simulink model "Multiplier"  (R2017b)
settings: Solver=ode45  StartTime=0.0  StopTime=10.0  RelTol=1e-3  EnableMultiTasking=on
libraries: hdlsllib x17
(part 1 of 3)
settings Model: Creator=you.r  LastModifiedBy=Ray
settings DataIOCC: LimitDataPoints=on  SaveFormat=Array
settings OptimizationCC: LifeSpan=inf
settings DebuggingCC: SolverPrmCheckMsg=warning  SFUnexpectedBacktrackingDiag=warning  SFNoUnconditionalDefaultTransitionDiag=warning  SFExecutionAtInitializationDiag=none
settings HardwareCC: ProdBitPerPointer=32  ProdBitPerSizeT=32  ProdBitPerPtrDiffT=32  ProdLargestAtomicFloat=None  ProdIntDivRoundTo=Undefined  ProdEndianess=Unspecified  ProdWordSize=32  ProdHWDeviceType=32-bit Generic
settings ModelReferenceCC: PropagateSignalLabelsOutOfModel=off
settings CodeAppCC: StateflowObjectComments=on
settings GRTTargetCC: TargetLangStandard=C89/C90 (ANSI)  GeneratePreprocessorConditionals=Disable all
settings ConfigComp: CovMetricSettings=dw  CovHtmlReporting=on  CovSaveCumulativeToWorkspaceVar=on  CovSaveSingleToWorkspaceVar=on  CovExternalEMLEnable=off  CovSFcnEnable=off

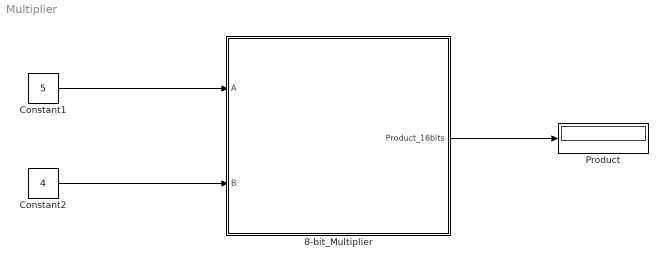
== system Multiplier ==
  8-bit_Multiplier : Subsystem
  Constant1 : Constant  Value=5  OutDataTypeStr=uint8  SampleTime=100
  Constant2 : Constant  Value=4  OutDataTypeStr=uint8  SampleTime=1
  Product : Display
  wires:
  8-bit_Multiplier/1(Product_16bits) -> Product/1
  Constant1/1 -> 8-bit_Multiplier/1(A)
  Constant2/1 -> 8-bit_Multiplier/2(B)

== system Multiplier/8-bit_Multiplier ==
  A : Inport  OutDataTypeStr=uint8
  B : Inport  Port=2  OutDataTypeStr=uint8
  Bit Concat : Subsystem
  Multiplier : Subsystem
  X Slicer : Subsystem
  X Slicer1 : Subsystem
  Product_16bits : Outport
  wires:
  B/1 -> X Slicer1/1(X)
  A/1 -> X Slicer/1(X)
  Bit Concat/1(out) -> Product_16bits/1
  Multiplier/1(P0) -> Bit Concat/16(In16)
  Multiplier/2(P1) -> Bit Concat/15(In15)
  Multiplier/3(P2) -> Bit Concat/14(In14)
  Multiplier/4(P3) -> Bit Concat/13(In13)
  Multiplier/5(P4) -> Bit Concat/12(In12)
  Multiplier/6(P5) -> Bit Concat/11(In11)
  Multiplier/7(P6) -> Bit Concat/10(In10)
  Multiplier/8(P7) -> Bit Concat/9(In9)
  Multiplier/9(P15) -> Bit Concat/1(In1)
  Multiplier/10(P14) -> Bit Concat/2(In2)
  Multiplier/11(P13) -> Bit Concat/3(In3)
  Multiplier/12(P12) -> Bit Concat/4(In4)
  Multiplier/13(P11) -> Bit Concat/5(In5)
  Multiplier/14(P10) -> Bit Concat/6(In6)
  Multiplier/15(P9) -> Bit Concat/7(In7)
  Multiplier/16(P8) -> Bit Concat/8(In8)
  X Slicer/1(Y0) -> Multiplier/8(A0)
  X Slicer/2(Y1) -> Multiplier/7(A1)
  X Slicer/3(Y2) -> Multiplier/6(A2)
  X Slicer/4(Y3) -> Multiplier/5(A3)
  X Slicer/5(Y4) -> Multiplier/4(A4)
  X Slicer/6(Y5) -> Multiplier/3(A5)
  X Slicer/7(Y6) -> Multiplier/2(A6)
  X Slicer/8(Y7) -> Multiplier/1(A7)
  X Slicer1/1(Y0) -> Multiplier/9(B0)
  X Slicer1/2(Y1) -> Multiplier/10(B1)
  X Slicer1/3(Y2) -> Multiplier/11(B2)
  X Slicer1/4(Y3) -> Multiplier/12(B3)
  X Slicer1/5(Y4) -> Multiplier/13(B4)
  X Slicer1/6(Y5) -> Multiplier/14(B5)
  X Slicer1/7(Y6) -> Multiplier/15(B6)
  X Slicer1/8(Y7) -> Multiplier/16(B7)

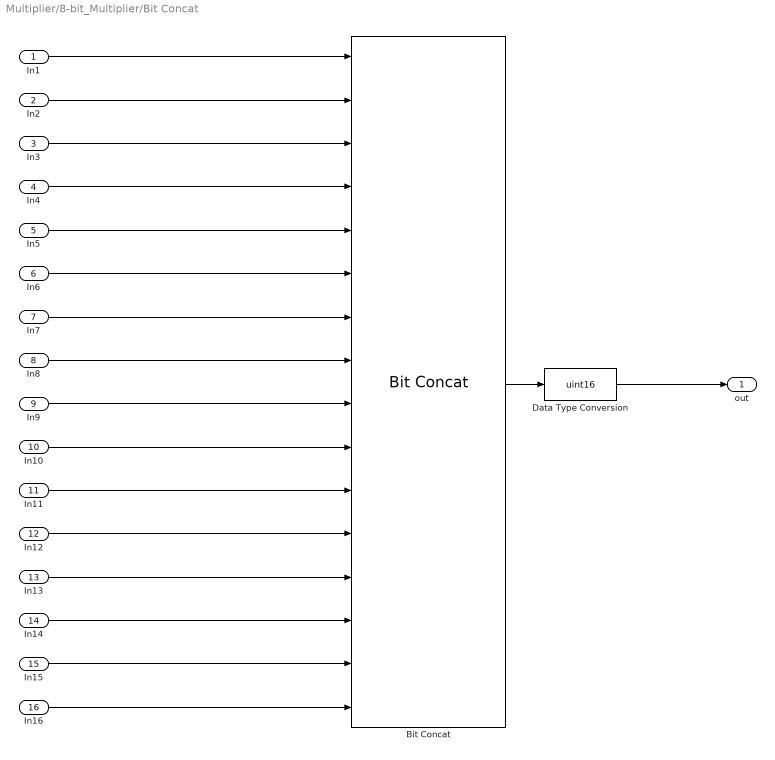
== system Multiplier/8-bit_Multiplier/Bit Concat ==
  In1 : Inport
  In2 : Inport  Port=2
  In3 : Inport  Port=3
  In4 : Inport  Port=4
  In5 : Inport  Port=5
  In6 : Inport  Port=6
  In7 : Inport  Port=7
  In8 : Inport  Port=8
  In9 : Inport  Port=9
  In10 : Inport  Port=10
  In11 : Inport  Port=11
  In12 : Inport  Port=12
  In13 : Inport  Port=13
  In14 : Inport  Port=14
  In15 : Inport  Port=15
  In16 : Inport  Port=16
  Bit Concat : hdlsllib/Logic and Bit Operations/Bit Concat  numInputs=16
      settings: SourceProductName=HDL Coder  SourceProductBaseCode=HD
  Data Type Conversion : DataTypeConversion  OutDataTypeStr=uint16
  out : Outport
  wires:
  Data Type Conversion/1 -> out/1
  Bit Concat/1 -> Data Type Conversion/1
  In13/1 -> Bit Concat/13
  In9/1 -> Bit Concat/9
  In10/1 -> Bit Concat/10
  In15/1 -> Bit Concat/15
  In1/1 -> Bit Concat/1
  In7/1 -> Bit Concat/7
  In2/1 -> Bit Concat/2
  In5/1 -> Bit Concat/5
  In11/1 -> Bit Concat/11
  In14/1 -> Bit Concat/14
  In12/1 -> Bit Concat/12
  In3/1 -> Bit Concat/3
  In4/1 -> Bit Concat/4
  In6/1 -> Bit Concat/6
  In16/1 -> Bit Concat/16
  In8/1 -> Bit Concat/8

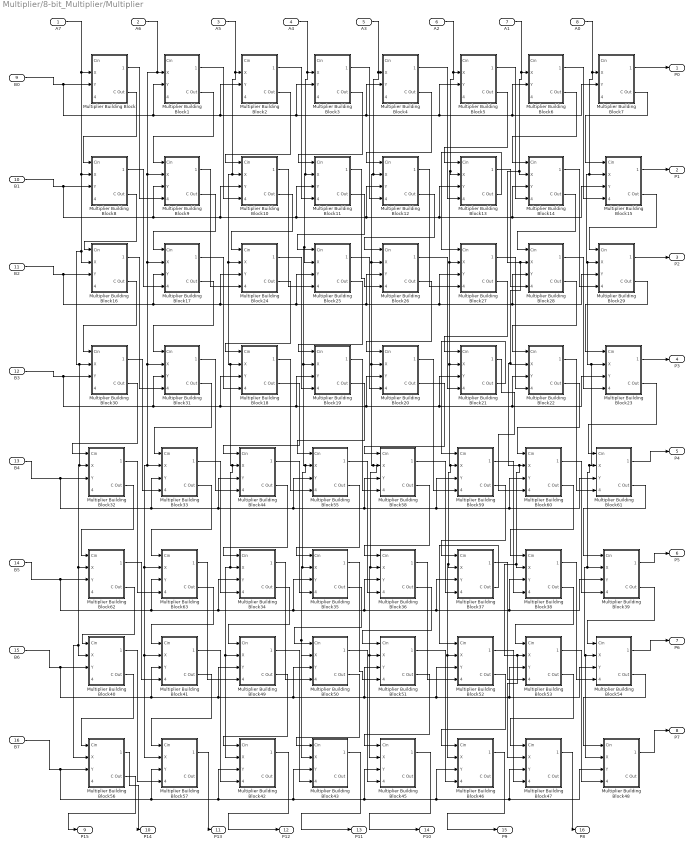
== system Multiplier/8-bit_Multiplier/Multiplier ==
  A7 : Inport
  A6 : Inport  Port=2
  A5 : Inport  Port=3
  A4 : Inport  Port=4
  A3 : Inport  Port=5
  A2 : Inport  Port=6
  A1 : Inport  Port=7
  A0 : Inport  Port=8
  B0 : Inport  Port=9  SampleTime=1
  B1 : Inport  Port=10  SampleTime=1
  B2 : Inport  Port=11  SampleTime=1
  B3 : Inport  Port=12  SampleTime=1
  B4 : Inport  Port=13  SampleTime=1
  B5 : Inport  Port=14  SampleTime=1
  B6 : Inport  Port=15  SampleTime=1
  B7 : Inport  Port=16  SampleTime=1
  Multiplier Building Block : Subsystem
  Multiplier Building Block1 : Subsystem
  Multiplier Building Block10 : Subsystem
  Multiplier Building Block11 : Subsystem
  Multiplier Building Block12 : Subsystem
  Multiplier Building Block13 : Subsystem
  Multiplier Building Block14 : Subsystem
  Multiplier Building Block15 : Subsystem
  Multiplier Building Block16 : Subsystem
  Multiplier Building Block17 : Subsystem
  Multiplier Building Block18 : Subsystem
  Multiplier Building Block19 : Subsystem
  Multiplier Building Block2 : Subsystem
  Multiplier Building Block20 : Subsystem
  Multiplier Building Block21 : Subsystem
  Multiplier Building Block22 : Subsystem
  Multiplier Building Block23 : Subsystem
  Multiplier Building Block24 : Subsystem
  Multiplier Building Block25 : Subsystem
  Multiplier Building Block26 : Subsystem
  Multiplier Building Block27 : Subsystem
  Multiplier Building Block28 : Subsystem
  Multiplier Building Block29 : Subsystem
  Multiplier Building Block3 : Subsystem
  Multiplier Building Block30 : Subsystem
  Multiplier Building Block31 : Subsystem
  Multiplier Building Block32 : Subsystem
  Multiplier Building Block33 : Subsystem
  Multiplier Building Block34 : Subsystem
  Multiplier Building Block35 : Subsystem
  Multiplier Building Block36 : Subsystem
  Multiplier Building Block37 : Subsystem
  Multiplier Building Block38 : Subsystem
  Multiplier Building Block39 : Subsystem
  Multiplier Building Block4 : Subsystem
  Multiplier Building Block40 : Subsystem
  Multiplier Building Block41 : Subsystem
  Multiplier Building Block42 : Subsystem
  Multiplier Building Block43 : Subsystem
  Multiplier Building Block44 : Subsystem
  Multiplier Building Block45 : Subsystem
  Multiplier Building Block46 : Subsystem
  Multiplier Building Block47 : Subsystem
  Multiplier Building Block48 : Subsystem
  Multiplier Building Block49 : Subsystem
  Multiplier Building Block5 : Subsystem
  Multiplier Building Block50 : Subsystem
  Multiplier Building Block51 : Subsystem
  Multiplier Building Block52 : Subsystem
  Multiplier Building Block53 : Subsystem
  Multiplier Building Block54 : Subsystem
  Multiplier Building Block55 : Subsystem
  Multiplier Building Block56 : Subsystem
  Multiplier Building Block57 : Subsystem
  Multiplier Building Block58 : Subsystem
  Multiplier Building Block59 : Subsystem
  Multiplier Building Block6 : Subsystem
  Multiplier Building Block60 : Subsystem
  Multiplier Building Block61 : Subsystem
  Multiplier Building Block62 : Subsystem
  Multiplier Building Block63 : Subsystem
  Multiplier Building Block7 : Subsystem
  Multiplier Building Block8 : Subsystem
  Multiplier Building Block9 : Subsystem
  P0 : Outport
  P1 : Outport  Port=2
  P2 : Outport  Port=3
  P3 : Outport  Port=4
  P4 : Outport  Port=5
  P5 : Outport  Port=6
  P6 : Outport  Port=7
  P7 : Outport  Port=8
  P15 : Outport  Port=9
  P14 : Outport  Port=10
  P13 : Outport  Port=11
  P12 : Outport  Port=12
  P11 : Outport  Port=13
  P10 : Outport  Port=14
  P9 : Outport  Port=15
  P8 : Outport  Port=16
  wires:
  Multiplier Building Block7/2(C Out) -> Multiplier Building Block15/1(Cin)
  Multiplier Building Block5/1(Sum Out) -> Multiplier Building Block14/4(Sum in)
  Multiplier Building Block6/1(Sum Out) -> Multiplier Building Block15/4(Sum in)
  Multiplier Building Block/2(C Out) -> Multiplier Building Block8/1(Cin)
  Multiplier Building Block/1(Sum Out) -> Multiplier Building Block9/4(Sum in)
  Multiplier Building Block5/2(C Out) -> Multiplier Building Block13/1(Cin)
  Multiplier Building Block2/2(C Out) -> Multiplier Building Block10/1(Cin)
  Multiplier Building Block6/2(C Out) -> Multiplier Building Block14/1(Cin)
  Multiplier Building Block4/1(Sum Out) -> Multiplier Building Block13/4(Sum in)
  Multiplier Building Block4/2(C Out) -> Multiplier Building Block12/1(Cin)
  Multiplier Building Block3/1(Sum Out) -> Multiplier Building Block12/4(Sum in)
  Multiplier Building Block3/2(C Out) -> Multiplier Building Block11/1(Cin)
  Multiplier Building Block2/1(Sum Out) -> Multiplier Building Block11/4(Sum in)
  Multiplier Building Block1/1(Sum Out) -> Multiplier Building Block10/4(Sum in)
  Multiplier Building Block1/2(C Out) -> Multiplier Building Block9/1(Cin)
  Multiplier Building Block7/1(Sum Out) -> P0/1
  B0/1 -> Multiplier Building Block3/3(Y), Multiplier Building Block7/3(Y), Multiplier Building Block6/3(Y), Multiplier Building Block5/3(Y), Multiplier Building Block4/3(Y), Multiplier Building Block2/3(Y), Multiplier Building Block1/3(Y), Multiplier Building Block/3(Y)
  Multiplier Building Block15/1(Sum Out) -> P1/1
  B1/1 -> Multiplier Building Block11/3(Y), Multiplier Building Block15/3(Y), Multiplier Building Block14/3(Y), Multiplier Building Block13/3(Y), Multiplier Building Block12/3(Y), Multiplier Building Block10/3(Y), Multiplier Building Block9/3(Y), Multiplier Building Block8/3(Y)
  Multiplier Building Block29/2(C Out) -> Multiplier Building Block23/1(Cin)
  Multiplier Building Block27/1(Sum Out) -> Multiplier Building Block22/4(Sum in)
  Multiplier Building Block28/1(Sum Out) -> Multiplier Building Block23/4(Sum in)
  Multiplier Building Block16/2(C Out) -> Multiplier Building Block30/1(Cin)
  Multiplier Building Block16/1(Sum Out) -> Multiplier Building Block31/4(Sum in)
  Multiplier Building Block27/2(C Out) -> Multiplier Building Block21/1(Cin)
  Multiplier Building Block24/2(C Out) -> Multiplier Building Block18/1(Cin)
  Multiplier Building Block28/2(C Out) -> Multiplier Building Block22/1(Cin)
  Multiplier Building Block26/1(Sum Out) -> Multiplier Building Block21/4(Sum in)
  Multiplier Building Block26/2(C Out) -> Multiplier Building Block20/1(Cin)
  Multiplier Building Block25/1(Sum Out) -> Multiplier Building Block20/4(Sum in)
  Multiplier Building Block25/2(C Out) -> Multiplier Building Block19/1(Cin)
  Multiplier Building Block24/1(Sum Out) -> Multiplier Building Block19/4(Sum in)
  Multiplier Building Block17/1(Sum Out) -> Multiplier Building Block18/4(Sum in)
  Multiplier Building Block17/2(C Out) -> Multiplier Building Block31/1(Cin)
  Multiplier Building Block29/1(Sum Out) -> P2/1
  B2/1 -> Multiplier Building Block25/3(Y), Multiplier Building Block29/3(Y), Multiplier Building Block28/3(Y), Multiplier Building Block27/3(Y), Multiplier Building Block26/3(Y), Multiplier Building Block24/3(Y), Multiplier Building Block17/3(Y), Multiplier Building Block16/3(Y)
  Multiplier Building Block23/1(Sum Out) -> P3/1
  B3/1 -> Multiplier Building Block19/3(Y), Multiplier Building Block23/3(Y), Multiplier Building Block22/3(Y), Multiplier Building Block21/3(Y), Multiplier Building Block20/3(Y), Multiplier Building Block18/3(Y), Multiplier Building Block31/3(Y), Multiplier Building Block30/3(Y)
  Multiplier Building Block15/2(C Out) -> Multiplier Building Block29/1(Cin)
  Multiplier Building Block14/1(Sum Out) -> Multiplier Building Block29/4(Sum in)
  Multiplier Building Block14/2(C Out) -> Multiplier Building Block28/1(Cin)
  Multiplier Building Block13/1(Sum Out) -> Multiplier Building Block28/4(Sum in)
  Multiplier Building Block13/2(C Out) -> Multiplier Building Block27/1(Cin)
  Multiplier Building Block12/1(Sum Out) -> Multiplier Building Block27/4(Sum in)
  Multiplier Building Block12/2(C Out) -> Multiplier Building Block26/1(Cin)
  Multiplier Building Block11/1(Sum Out) -> Multiplier Building Block26/4(Sum in)
  Multiplier Building Block11/2(C Out) -> Multiplier Building Block25/1(Cin)
  Multiplier Building Block10/1(Sum Out) -> Multiplier Building Block25/4(Sum in)
  Multiplier Building Block10/2(C Out) -> Multiplier Building Block24/1(Cin)
  Multiplier Building Block9/1(Sum Out) -> Multiplier Building Block24/4(Sum in)
  Multiplier Building Block9/2(C Out) -> Multiplier Building Block17/1(Cin)
  Multiplier Building Block8/1(Sum Out) -> Multiplier Building Block17/4(Sum in)
  Multiplier Building Block8/2(C Out) -> Multiplier Building Block16/1(Cin)
  Multiplier Building Block61/2(C Out) -> Multiplier Building Block39/1(Cin)
  Multiplier Building Block59/1(Sum Out) -> Multiplier Building Block38/4(Sum in)
  Multiplier Building Block60/1(Sum Out) -> Multiplier Building Block39/4(Sum in)
  Multiplier Building Block32/2(C Out) -> Multiplier Building Block62/1(Cin)
  Multiplier Building Block32/1(Sum Out) -> Multiplier Building Block63/4(Sum in)
  Multiplier Building Block59/2(C Out) -> Multiplier Building Block37/1(Cin)
  Multiplier Building Block44/2(C Out) -> Multiplier Building Block34/1(Cin)
  Multiplier Building Block60/2(C Out) -> Multiplier Building Block38/1(Cin)
  Multiplier Building Block58/1(Sum Out) -> Multiplier Building Block37/4(Sum in)
  Multiplier Building Block58/2(C Out) -> Multiplier Building Block36/1(Cin)
  Multiplier Building Block55/1(Sum Out) -> Multiplier Building Block36/4(Sum in)
  Multiplier Building Block55/2(C Out) -> Multiplier Building Block35/1(Cin)
  Multiplier Building Block44/1(Sum Out) -> Multiplier Building Block35/4(Sum in)
  Multiplier Building Block33/1(Sum Out) -> Multiplier Building Block34/4(Sum in)
  Multiplier Building Block33/2(C Out) -> Multiplier Building Block63/1(Cin)
  A7/1 -> Multiplier Building Block56/2(X), Multiplier Building Block40/2(X), Multiplier Building Block62/2(X), Multiplier Building Block32/2(X), Multiplier Building Block30/2(X), Multiplier Building Block16/2(X), Multiplier Building Block8/2(X), Multiplier Building Block/2(X)
  A6/1 -> Multiplier Building Block9/2(X), Multiplier Building Block31/2(X), Multiplier Building Block33/2(X), Multiplier Building Block63/2(X), Multiplier Building Block57/2(X), Multiplier Building Block41/2(X), Multiplier Building Block17/2(X), Multiplier Building Block1/2(X)
  A5/1 -> Multiplier Building Block10/2(X), Multiplier Building Block34/2(X), Multiplier Building Block42/2(X), Multiplier Building Block49/2(X), Multiplier Building Block44/2(X), Multiplier Building Block18/2(X), Multiplier Building Block24/2(X), Multiplier Building Block2/2(X)
  A4/1 -> Multiplier Building Block11/2(X), Multiplier Building Block19/2(X), Multiplier Building Block35/2(X), Multiplier Building Block43/2(X), Multiplier Building Block50/2(X), Multiplier Building Block55/2(X), Multiplier Building Block25/2(X), Multiplier Building Block3/2(X)
  A3/1 -> Multiplier Building Block12/2(X), Multiplier Building Block20/2(X), Multiplier Building Block36/2(X), Multiplier Building Block45/2(X), Multiplier Building Block51/2(X), Multiplier Building Block58/2(X), Multiplier Building Block26/2(X), Multiplier Building Block4/2(X)
  A2/1 -> Multiplier Building Block21/2(X), Multiplier Building Block46/2(X), Multiplier Building Block52/2(X), Multiplier Building Block37/2(X), Multiplier Building Block59/2(X), Multiplier Building Block27/2(X), Multiplier Building Block13/2(X), Multiplier Building Block5/2(X)
  A0/1 -> Multiplier Building Block29/2(X), Multiplier Building Block54/2(X), Multiplier Building Block48/2(X), Multiplier Building Block39/2(X), Multiplier Building Block61/2(X), Multiplier Building Block23/2(X), Multiplier Building Block15/2(X), Multiplier Building Block7/2(X)
  A1/1 -> Multiplier Building Block47/2(X), Multiplier Building Block53/2(X), Multiplier Building Block38/2(X), Multiplier Building Block60/2(X), Multiplier Building Block22/2(X), Multiplier Building Block28/2(X), Multiplier Building Block14/2(X), Multiplier Building Block6/2(X)
  Multiplier Building Block61/1(Sum Out) -> P4/1
  B4/1 -> Multiplier Building Block55/3(Y), Multiplier Building Block61/3(Y), Multiplier Building Block60/3(Y), Multiplier Building Block59/3(Y), Multiplier Building Block58/3(Y), Multiplier Building Block44/3(Y), Multiplier Building Block33/3(Y), Multiplier Building Block32/3(Y)
  Multiplier Building Block39/1(Sum Out) -> P5/1
  B5/1 -> Multiplier Building Block35/3(Y), Multiplier Building Block39/3(Y), Multiplier Building Block38/3(Y), Multiplier Building Block37/3(Y), Multiplier Building Block36/3(Y), Multiplier Building Block34/3(Y), Multiplier Building Block63/3(Y), Multiplier Building Block62/3(Y)
  Multiplier Building Block54/2(C Out) -> Multiplier Building Block48/1(Cin)
  Multiplier Building Block52/1(Sum Out) -> Multiplier Building Block47/4(Sum in)
  Multiplier Building Block53/1(Sum Out) -> Multiplier Building Block48/4(Sum in)
  Multiplier Building Block40/2(C Out) -> Multiplier Building Block56/1(Cin)
  Multiplier Building Block40/1(Sum Out) -> Multiplier Building Block57/4(Sum in)
  Multiplier Building Block52/2(C Out) -> Multiplier Building Block46/1(Cin)
  Multiplier Building Block49/2(C Out) -> Multiplier Building Block42/1(Cin)
  Multiplier Building Block53/2(C Out) -> Multiplier Building Block47/1(Cin)
  Multiplier Building Block51/1(Sum Out) -> Multiplier Building Block46/4(Sum in)
  Multiplier Building Block51/2(C Out) -> Multiplier Building Block45/1(Cin)
  Multiplier Building Block50/1(Sum Out) -> Multiplier Building Block45/4(Sum in)
  Multiplier Building Block50/2(C Out) -> Multiplier Building Block43/1(Cin)
  Multiplier Building Block49/1(Sum Out) -> Multiplier Building Block43/4(Sum in)
  Multiplier Building Block41/1(Sum Out) -> Multiplier Building Block42/4(Sum in)
  Multiplier Building Block41/2(C Out) -> Multiplier Building Block57/1(Cin)
  Multiplier Building Block54/1(Sum Out) -> P6/1
  B6/1 -> Multiplier Building Block50/3(Y), Multiplier Building Block54/3(Y), Multiplier Building Block53/3(Y), Multiplier Building Block52/3(Y), Multiplier Building Block51/3(Y), Multiplier Building Block49/3(Y), Multiplier Building Block41/3(Y), Multiplier Building Block40/3(Y)
  Multiplier Building Block48/1(Sum Out) -> P7/1
  B7/1 -> Multiplier Building Block43/3(Y), Multiplier Building Block48/3(Y), Multiplier Building Block47/3(Y), Multiplier Building Block46/3(Y), Multiplier Building Block45/3(Y), Multiplier Building Block42/3(Y), Multiplier Building Block57/3(Y), Multiplier Building Block56/3(Y)
  Multiplier Building Block39/2(C Out) -> Multiplier Building Block54/1(Cin)
  Multiplier Building Block38/1(Sum Out) -> Multiplier Building Block54/4(Sum in)
  Multiplier Building Block38/2(C Out) -> Multiplier Building Block53/1(Cin)
  Multiplier Building Block37/1(Sum Out) -> Multiplier Building Block53/4(Sum in)
  Multiplier Building Block37/2(C Out) -> Multiplier Building Block52/1(Cin)
  Multiplier Building Block36/1(Sum Out) -> Multiplier Building Block52/4(Sum in)
  Multiplier Building Block36/2(C Out) -> Multiplier Building Block51/1(Cin)
  Multiplier Building Block35/1(Sum Out) -> Multiplier Building Block51/4(Sum in)
  Multiplier Building Block35/2(C Out) -> Multiplier Building Block50/1(Cin)
  Multiplier Building Block34/1(Sum Out) -> Multiplier Building Block50/4(Sum in)
  Multiplier Building Block34/2(C Out) -> Multiplier Building Block49/1(Cin)
  Multiplier Building Block63/1(Sum Out) -> Multiplier Building Block49/4(Sum in)
  Multiplier Building Block63/2(C Out) -> Multiplier Building Block41/1(Cin)
  Multiplier Building Block62/1(Sum Out) -> Multiplier Building Block41/4(Sum in)
  Multiplier Building Block62/2(C Out) -> Multiplier Building Block40/1(Cin)
  Multiplier Building Block23/2(C Out) -> Multiplier Building Block61/1(Cin)
  Multiplier Building Block22/1(Sum Out) -> Multiplier Building Block61/4(Sum in)
  Multiplier Building Block22/2(C Out) -> Multiplier Building Block60/1(Cin)
  Multiplier Building Block21/1(Sum Out) -> Multiplier Building Block60/4(Sum in)
  Multiplier Building Block21/2(C Out) -> Multiplier Building Block59/1(Cin)
  Multiplier Building Block20/1(Sum Out) -> Multiplier Building Block59/4(Sum in)
  Multiplier Building Block20/2(C Out) -> Multiplier Building Block58/1(Cin)
  Multiplier Building Block19/1(Sum Out) -> Multiplier Building Block58/4(Sum in)
  Multiplier Building Block19/2(C Out) -> Multiplier Building Block55/1(Cin)
  Multiplier Building Block18/1(Sum Out) -> Multiplier Building Block55/4(Sum in)
  Multiplier Building Block18/2(C Out) -> Multiplier Building Block44/1(Cin)
  Multiplier Building Block31/1(Sum Out) -> Multiplier Building Block44/4(Sum in)
  Multiplier Building Block31/2(C Out) -> Multiplier Building Block33/1(Cin)
  Multiplier Building Block30/1(Sum Out) -> Multiplier Building Block33/4(Sum in)
  Multiplier Building Block30/2(C Out) -> Multiplier Building Block32/1(Cin)
  Multiplier Building Block56/2(C Out) -> P15/1
  Multiplier Building Block56/1(Sum Out) -> P14/1
  Multiplier Building Block57/1(Sum Out) -> P13/1
  Multiplier Building Block42/1(Sum Out) -> P12/1
  Multiplier Building Block43/1(Sum Out) -> P11/1
  Multiplier Building Block45/1(Sum Out) -> P10/1
  Multiplier Building Block46/1(Sum Out) -> P9/1
  Multiplier Building Block47/1(Sum Out) -> P8/1

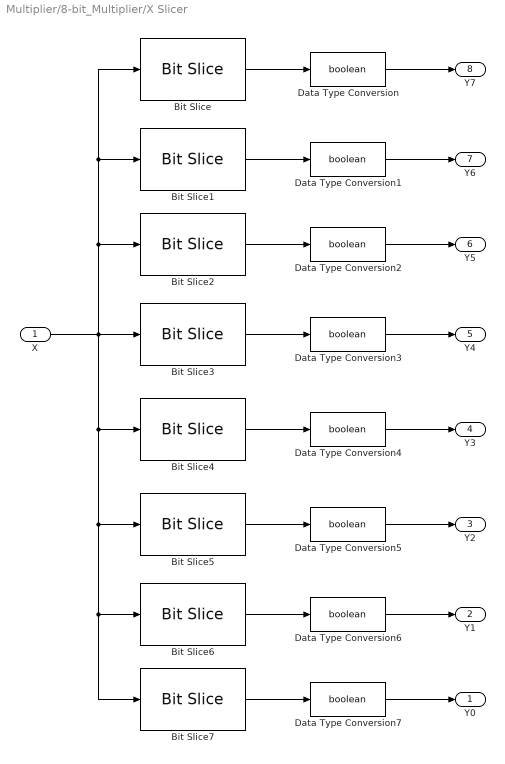
== system Multiplier/8-bit_Multiplier/X Slicer ==
  X : Inport  OutDataTypeStr=uint8  SampleTime=1
  Bit Slice : hdlsllib/Logic and Bit Operations/Bit Slice  lidx=7  ridx=7
  Bit Slice1 : hdlsllib/Logic and Bit Operations/Bit Slice  lidx=6  ridx=6
  Bit Slice2 : hdlsllib/Logic and Bit Operations/Bit Slice  lidx=5  ridx=5
  Bit Slice3 : hdlsllib/Logic and Bit Operations/Bit Slice  lidx=4  ridx=4
  Bit Slice4 : hdlsllib/Logic and Bit Operations/Bit Slice  lidx=3  ridx=3
  Bit Slice5 : hdlsllib/Logic and Bit Operations/Bit Slice  lidx=2  ridx=2
  Bit Slice6 : hdlsllib/Logic and Bit Operations/Bit Slice  lidx=1  ridx=1
  Bit Slice7 : hdlsllib/Logic and Bit Operations/Bit Slice  lidx=0  ridx=0
  Data Type Conversion{,1..7} (8 alike) : DataTypeConversion  OutDataTypeStr=boolean
  Y0 : Outport
  Y1 : Outport  Port=2
  Y2 : Outport  Port=3
  Y3 : Outport  Port=4
  Y4 : Outport  Port=5
  Y5 : Outport  Port=6
  Y6 : Outport  Port=7
  Y7 : Outport  Port=8
  wires:
  X/1 -> Bit Slice4/1, Bit Slice5/1, Bit Slice6/1, Bit Slice7/1, Bit Slice3/1, Bit Slice2/1, Bit Slice1/1, Bit Slice/1
  Data Type Conversion/1 -> Y7/1
  Data Type Conversion1/1 -> Y6/1
  Bit Slice2/1 -> Data Type Conversion2/1
  Bit Slice3/1 -> Data Type Conversion3/1
  Bit Slice4/1 -> Data Type Conversion4/1
  Data Type Conversion6/1 -> Y1/1
  Bit Slice/1 -> Data Type Conversion/1
  Bit Slice1/1 -> Data Type Conversion1/1
  Bit Slice6/1 -> Data Type Conversion6/1
  Data Type Conversion7/1 -> Y0/1
  Bit Slice7/1 -> Data Type Conversion7/1
  Bit Slice5/1 -> Data Type Conversion5/1
  Data Type Conversion2/1 -> Y5/1
  Data Type Conversion3/1 -> Y4/1
  Data Type Conversion4/1 -> Y3/1
  Data Type Conversion5/1 -> Y2/1

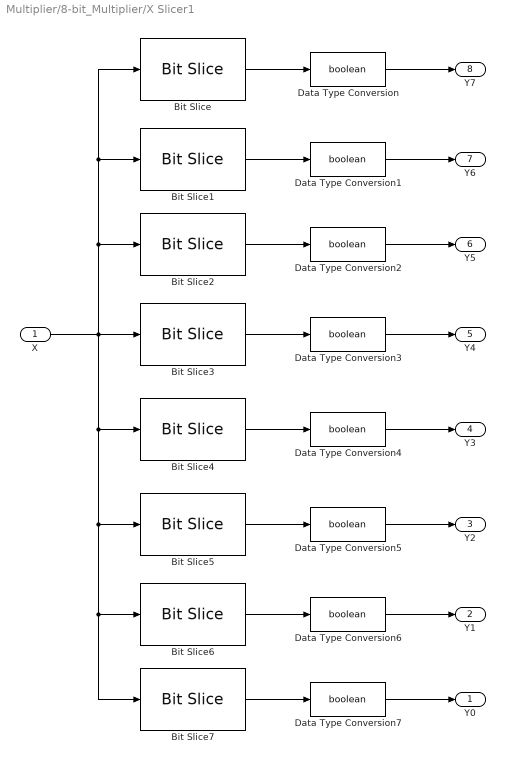
== system Multiplier/8-bit_Multiplier/X Slicer1 ==
  X : Inport  OutDataTypeStr=uint8  SampleTime=1
  Bit Slice : hdlsllib/Logic and Bit Operations/Bit Slice  lidx=7  ridx=7
  Bit Slice1 : hdlsllib/Logic and Bit Operations/Bit Slice  lidx=6  ridx=6
  Bit Slice2 : hdlsllib/Logic and Bit Operations/Bit Slice  lidx=5  ridx=5
  Bit Slice3 : hdlsllib/Logic and Bit Operations/Bit Slice  lidx=4  ridx=4
  Bit Slice4 : hdlsllib/Logic and Bit Operations/Bit Slice  lidx=3  ridx=3
  Bit Slice5 : hdlsllib/Logic and Bit Operations/Bit Slice  lidx=2  ridx=2
  Bit Slice6 : hdlsllib/Logic and Bit Operations/Bit Slice  lidx=1  ridx=1
  Bit Slice7 : hdlsllib/Logic and Bit Operations/Bit Slice  lidx=0  ridx=0
  Data Type Conversion{,1..7} (8 alike) : DataTypeConversion  OutDataTypeStr=boolean
  Y0 : Outport
  Y1 : Outport  Port=2
  Y2 : Outport  Port=3
  Y3 : Outport  Port=4
  Y4 : Outport  Port=5
  Y5 : Outport  Port=6
  Y6 : Outport  Port=7
  Y7 : Outport  Port=8
  wires:
  X/1 -> Bit Slice4/1, Bit Slice5/1, Bit Slice6/1, Bit Slice7/1, Bit Slice3/1, Bit Slice2/1, Bit Slice1/1, Bit Slice/1
  Data Type Conversion/1 -> Y7/1
  Data Type Conversion1/1 -> Y6/1
  Bit Slice2/1 -> Data Type Conversion2/1
  Bit Slice3/1 -> Data Type Conversion3/1
  Bit Slice4/1 -> Data Type Conversion4/1
  Data Type Conversion6/1 -> Y1/1
  Bit Slice/1 -> Data Type Conversion/1
  Bit Slice1/1 -> Data Type Conversion1/1
  Bit Slice6/1 -> Data Type Conversion6/1
  Data Type Conversion7/1 -> Y0/1
  Bit Slice7/1 -> Data Type Conversion7/1
  Bit Slice5/1 -> Data Type Conversion5/1
  Data Type Conversion2/1 -> Y5/1
  Data Type Conversion3/1 -> Y4/1
  Data Type Conversion4/1 -> Y3/1
  Data Type Conversion5/1 -> Y2/1

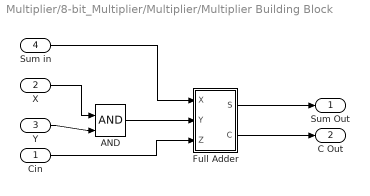
== system Multiplier/8-bit_Multiplier/Multiplier/Multiplier Building Block ==
  Cin : Inport
  X : Inport  Port=2
  Y : Inport  Port=3
  Sum in : Inport  Port=4
  AND : Logic  IconShape=distinctive  AllPortsSameDT=off  OutDataTypeStr=boolean
  Full Adder : Subsystem
  Sum Out : Outport
  C Out : Outport  Port=2
  wires:
  Cin/1 -> Full Adder/3(Z)
  Sum in/1 -> Full Adder/1(X)
  AND/1 -> Full Adder/2(Y)
  Full Adder/1(S) -> Sum Out/1
  Y/1 -> AND/2
  X/1 -> AND/1
  Full Adder/2(C) -> C Out/1

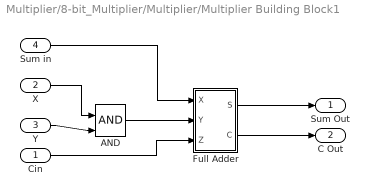
== system Multiplier/8-bit_Multiplier/Multiplier/Multiplier Building Block1 ==
  Cin : Inport
  X : Inport  Port=2
  Y : Inport  Port=3
  Sum in : Inport  Port=4
  AND : Logic  IconShape=distinctive  AllPortsSameDT=off  OutDataTypeStr=boolean
  Full Adder : Subsystem
  Sum Out : Outport
  C Out : Outport  Port=2
  wires:
  Cin/1 -> Full Adder/3(Z)
  Sum in/1 -> Full Adder/1(X)
  AND/1 -> Full Adder/2(Y)
  Full Adder/1(S) -> Sum Out/1
  Y/1 -> AND/2
  X/1 -> AND/1
  Full Adder/2(C) -> C Out/1

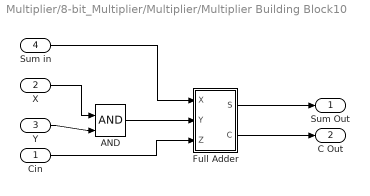
== system Multiplier/8-bit_Multiplier/Multiplier/Multiplier Building Block10 ==
  Cin : Inport
  X : Inport  Port=2
  Y : Inport  Port=3
  Sum in : Inport  Port=4
  AND : Logic  IconShape=distinctive  AllPortsSameDT=off  OutDataTypeStr=boolean
  Full Adder : Subsystem
  Sum Out : Outport
  C Out : Outport  Port=2
  wires:
  Cin/1 -> Full Adder/3(Z)
  Sum in/1 -> Full Adder/1(X)
  AND/1 -> Full Adder/2(Y)
  Full Adder/1(S) -> Sum Out/1
  Y/1 -> AND/2
  X/1 -> AND/1
  Full Adder/2(C) -> C Out/1

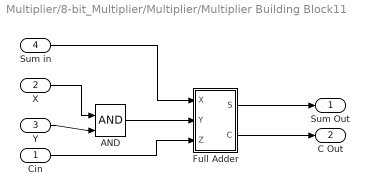
== system Multiplier/8-bit_Multiplier/Multiplier/Multiplier Building Block11 ==
  Cin : Inport
  X : Inport  Port=2
  Y : Inport  Port=3
  Sum in : Inport  Port=4
  AND : Logic  IconShape=distinctive  AllPortsSameDT=off  OutDataTypeStr=boolean
  Full Adder : Subsystem
  Sum Out : Outport
  C Out : Outport  Port=2
  wires:
  Cin/1 -> Full Adder/3(Z)
  Sum in/1 -> Full Adder/1(X)
  AND/1 -> Full Adder/2(Y)
  Full Adder/1(S) -> Sum Out/1
  Y/1 -> AND/2
  X/1 -> AND/1
  Full Adder/2(C) -> C Out/1

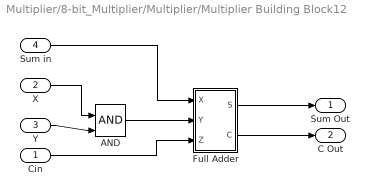
== system Multiplier/8-bit_Multiplier/Multiplier/Multiplier Building Block12 ==
  Cin : Inport
  X : Inport  Port=2
  Y : Inport  Port=3
  Sum in : Inport  Port=4
  AND : Logic  IconShape=distinctive  AllPortsSameDT=off  OutDataTypeStr=boolean
  Full Adder : Subsystem
  Sum Out : Outport
  C Out : Outport  Port=2
  wires:
  Cin/1 -> Full Adder/3(Z)
  Sum in/1 -> Full Adder/1(X)
  AND/1 -> Full Adder/2(Y)
  Full Adder/1(S) -> Sum Out/1
  Y/1 -> AND/2
  X/1 -> AND/1
  Full Adder/2(C) -> C Out/1

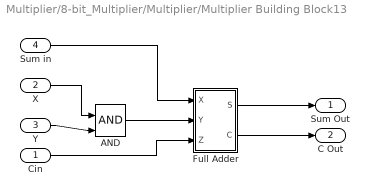
== system Multiplier/8-bit_Multiplier/Multiplier/Multiplier Building Block13 ==
  Cin : Inport
  X : Inport  Port=2
  Y : Inport  Port=3
  Sum in : Inport  Port=4
  AND : Logic  IconShape=distinctive  AllPortsSameDT=off  OutDataTypeStr=boolean
  Full Adder : Subsystem
  Sum Out : Outport
  C Out : Outport  Port=2
  wires:
  Cin/1 -> Full Adder/3(Z)
  Sum in/1 -> Full Adder/1(X)
  AND/1 -> Full Adder/2(Y)
  Full Adder/1(S) -> Sum Out/1
  Y/1 -> AND/2
  X/1 -> AND/1
  Full Adder/2(C) -> C Out/1

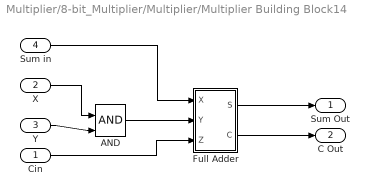
== system Multiplier/8-bit_Multiplier/Multiplier/Multiplier Building Block14 ==
  Cin : Inport
  X : Inport  Port=2
  Y : Inport  Port=3
  Sum in : Inport  Port=4
  AND : Logic  IconShape=distinctive  AllPortsSameDT=off  OutDataTypeStr=boolean
  Full Adder : Subsystem
  Sum Out : Outport
  C Out : Outport  Port=2
  wires:
  Cin/1 -> Full Adder/3(Z)
  Sum in/1 -> Full Adder/1(X)
  AND/1 -> Full Adder/2(Y)
  Full Adder/1(S) -> Sum Out/1
  Y/1 -> AND/2
  X/1 -> AND/1
  Full Adder/2(C) -> C Out/1

== system Multiplier/8-bit_Multiplier/Multiplier/Multiplier Building Block15 ==
  Cin : Inport
  X : Inport  Port=2
  Y : Inport  Port=3
  Sum in : Inport  Port=4
  AND : Logic  IconShape=distinctive  AllPortsSameDT=off  OutDataTypeStr=boolean
  Full Adder : Subsystem
  Sum Out : Outport
  C Out : Outport  Port=2
  wires:
  Cin/1 -> Full Adder/3(Z)
  Sum in/1 -> Full Adder/1(X)
  AND/1 -> Full Adder/2(Y)
  Full Adder/1(S) -> Sum Out/1
  Y/1 -> AND/2
  X/1 -> AND/1
  Full Adder/2(C) -> C Out/1

== system Multiplier/8-bit_Multiplier/Multiplier/Multiplier Building Block16 ==
  Cin : Inport
  X : Inport  Port=2
  Y : Inport  Port=3
  Sum in : Inport  Port=4
  AND : Logic  IconShape=distinctive  AllPortsSameDT=off  OutDataTypeStr=boolean
  Full Adder : Subsystem
  Sum Out : Outport
  C Out : Outport  Port=2
  wires:
  Cin/1 -> Full Adder/3(Z)
  Sum in/1 -> Full Adder/1(X)
  AND/1 -> Full Adder/2(Y)
  Full Adder/1(S) -> Sum Out/1
  Y/1 -> AND/2
  X/1 -> AND/1
  Full Adder/2(C) -> C Out/1

== system Multiplier/8-bit_Multiplier/Multiplier/Multiplier Building Block17 ==
  Cin : Inport
  X : Inport  Port=2
  Y : Inport  Port=3
  Sum in : Inport  Port=4
  AND : Logic  IconShape=distinctive  AllPortsSameDT=off  OutDataTypeStr=boolean
  Full Adder : Subsystem
  Sum Out : Outport
  C Out : Outport  Port=2
  wires:
  Cin/1 -> Full Adder/3(Z)
  Sum in/1 -> Full Adder/1(X)
  AND/1 -> Full Adder/2(Y)
  Full Adder/1(S) -> Sum Out/1
  Y/1 -> AND/2
  X/1 -> AND/1
  Full Adder/2(C) -> C Out/1

== system Multiplier/8-bit_Multiplier/Multiplier/Multiplier Building Block18 ==
  Cin : Inport
  X : Inport  Port=2
  Y : Inport  Port=3
  Sum in : Inport  Port=4
  AND : Logic  IconShape=distinctive  AllPortsSameDT=off  OutDataTypeStr=boolean
  Full Adder : Subsystem
  Sum Out : Outport
  C Out : Outport  Port=2
  wires:
  Cin/1 -> Full Adder/3(Z)
  Sum in/1 -> Full Adder/1(X)
  AND/1 -> Full Adder/2(Y)
  Full Adder/1(S) -> Sum Out/1
  Y/1 -> AND/2
  X/1 -> AND/1
  Full Adder/2(C) -> C Out/1

== system Multiplier/8-bit_Multiplier/Multiplier/Multiplier Building Block19 ==
  Cin : Inport
  X : Inport  Port=2
  Y : Inport  Port=3
  Sum in : Inport  Port=4
  AND : Logic  IconShape=distinctive  AllPortsSameDT=off  OutDataTypeStr=boolean
  Full Adder : Subsystem
  Sum Out : Outport
  C Out : Outport  Port=2
  wires:
  Cin/1 -> Full Adder/3(Z)
  Sum in/1 -> Full Adder/1(X)
  AND/1 -> Full Adder/2(Y)
  Full Adder/1(S) -> Sum Out/1
  Y/1 -> AND/2
  X/1 -> AND/1
  Full Adder/2(C) -> C Out/1

== system Multiplier/8-bit_Multiplier/Multiplier/Multiplier Building Block2 ==
  Cin : Inport
  X : Inport  Port=2
  Y : Inport  Port=3
  Sum in : Inport  Port=4
  AND : Logic  IconShape=distinctive  AllPortsSameDT=off  OutDataTypeStr=boolean
  Full Adder : Subsystem
  Sum Out : Outport
  C Out : Outport  Port=2
  wires:
  Cin/1 -> Full Adder/3(Z)
  Sum in/1 -> Full Adder/1(X)
  AND/1 -> Full Adder/2(Y)
  Full Adder/1(S) -> Sum Out/1
  Y/1 -> AND/2
  X/1 -> AND/1
  Full Adder/2(C) -> C Out/1

== system Multiplier/8-bit_Multiplier/Multiplier/Multiplier Building Block20 ==
  Cin : Inport
  X : Inport  Port=2
  Y : Inport  Port=3
  Sum in : Inport  Port=4
  AND : Logic  IconShape=distinctive  AllPortsSameDT=off  OutDataTypeStr=boolean
  Full Adder : Subsystem
  Sum Out : Outport
  C Out : Outport  Port=2
  wires:
  Cin/1 -> Full Adder/3(Z)
  Sum in/1 -> Full Adder/1(X)
  AND/1 -> Full Adder/2(Y)
  Full Adder/1(S) -> Sum Out/1
  Y/1 -> AND/2
  X/1 -> AND/1
  Full Adder/2(C) -> C Out/1

== system Multiplier/8-bit_Multiplier/Multiplier/Multiplier Building Block21 ==
  Cin : Inport
  X : Inport  Port=2
  Y : Inport  Port=3
  Sum in : Inport  Port=4
  AND : Logic  IconShape=distinctive  AllPortsSameDT=off  OutDataTypeStr=boolean
  Full Adder : Subsystem
  Sum Out : Outport
  C Out : Outport  Port=2
  wires:
  Cin/1 -> Full Adder/3(Z)
  Sum in/1 -> Full Adder/1(X)
  AND/1 -> Full Adder/2(Y)
  Full Adder/1(S) -> Sum Out/1
  Y/1 -> AND/2
  X/1 -> AND/1
  Full Adder/2(C) -> C Out/1

== system Multiplier/8-bit_Multiplier/Multiplier/Multiplier Building Block22 ==
  Cin : Inport
  X : Inport  Port=2
  Y : Inport  Port=3
  Sum in : Inport  Port=4
  AND : Logic  IconShape=distinctive  AllPortsSameDT=off  OutDataTypeStr=boolean
  Full Adder : Subsystem
  Sum Out : Outport
  C Out : Outport  Port=2
  wires:
  Cin/1 -> Full Adder/3(Z)
  Sum in/1 -> Full Adder/1(X)
  AND/1 -> Full Adder/2(Y)
  Full Adder/1(S) -> Sum Out/1
  Y/1 -> AND/2
  X/1 -> AND/1
  Full Adder/2(C) -> C Out/1

== system Multiplier/8-bit_Multiplier/Multiplier/Multiplier Building Block23 ==
  Cin : Inport
  X : Inport  Port=2
  Y : Inport  Port=3
  Sum in : Inport  Port=4
  AND : Logic  IconShape=distinctive  AllPortsSameDT=off  OutDataTypeStr=boolean
  Full Adder : Subsystem
  Sum Out : Outport
  C Out : Outport  Port=2
  wires:
  Cin/1 -> Full Adder/3(Z)
  Sum in/1 -> Full Adder/1(X)
  AND/1 -> Full Adder/2(Y)
  Full Adder/1(S) -> Sum Out/1
  Y/1 -> AND/2
  X/1 -> AND/1
  Full Adder/2(C) -> C Out/1

== system Multiplier/8-bit_Multiplier/Multiplier/Multiplier Building Block24 ==
  Cin : Inport
  X : Inport  Port=2
  Y : Inport  Port=3
  Sum in : Inport  Port=4
  AND : Logic  IconShape=distinctive  AllPortsSameDT=off  OutDataTypeStr=boolean
  Full Adder : Subsystem
  Sum Out : Outport
  C Out : Outport  Port=2
  wires:
  Cin/1 -> Full Adder/3(Z)
  Sum in/1 -> Full Adder/1(X)
  AND/1 -> Full Adder/2(Y)
  Full Adder/1(S) -> Sum Out/1
  Y/1 -> AND/2
  X/1 -> AND/1
  Full Adder/2(C) -> C Out/1

== system Multiplier/8-bit_Multiplier/Multiplier/Multiplier Building Block25 ==
  Cin : Inport
  X : Inport  Port=2
  Y : Inport  Port=3
  Sum in : Inport  Port=4
  AND : Logic  IconShape=distinctive  AllPortsSameDT=off  OutDataTypeStr=boolean
  Full Adder : Subsystem
  Sum Out : Outport
  C Out : Outport  Port=2
  wires:
  Cin/1 -> Full Adder/3(Z)
  Sum in/1 -> Full Adder/1(X)
  AND/1 -> Full Adder/2(Y)
  Full Adder/1(S) -> Sum Out/1
  Y/1 -> AND/2
  X/1 -> AND/1
  Full Adder/2(C) -> C Out/1

== system Multiplier/8-bit_Multiplier/Multiplier/Multiplier Building Block26 ==
  Cin : Inport
  X : Inport  Port=2
  Y : Inport  Port=3
  Sum in : Inport  Port=4
  AND : Logic  IconShape=distinctive  AllPortsSameDT=off  OutDataTypeStr=boolean
  Full Adder : Subsystem
  Sum Out : Outport
  C Out : Outport  Port=2
  wires:
  Cin/1 -> Full Adder/3(Z)
  Sum in/1 -> Full Adder/1(X)
  AND/1 -> Full Adder/2(Y)
  Full Adder/1(S) -> Sum Out/1
  Y/1 -> AND/2
  X/1 -> AND/1
  Full Adder/2(C) -> C Out/1

== system Multiplier/8-bit_Multiplier/Multiplier/Multiplier Building Block27 ==
  Cin : Inport
  X : Inport  Port=2
  Y : Inport  Port=3
  Sum in : Inport  Port=4
  AND : Logic  IconShape=distinctive  AllPortsSameDT=off  OutDataTypeStr=boolean
  Full Adder : Subsystem
  Sum Out : Outport
  C Out : Outport  Port=2
  wires:
  Cin/1 -> Full Adder/3(Z)
  Sum in/1 -> Full Adder/1(X)
  AND/1 -> Full Adder/2(Y)
  Full Adder/1(S) -> Sum Out/1
  Y/1 -> AND/2
  X/1 -> AND/1
  Full Adder/2(C) -> C Out/1

== system Multiplier/8-bit_Multiplier/Multiplier/Multiplier Building Block28 ==
  Cin : Inport
  X : Inport  Port=2
  Y : Inport  Port=3
  Sum in : Inport  Port=4
  AND : Logic  IconShape=distinctive  AllPortsSameDT=off  OutDataTypeStr=boolean
  Full Adder : Subsystem
  Sum Out : Outport
  C Out : Outport  Port=2
  wires:
  Cin/1 -> Full Adder/3(Z)
  Sum in/1 -> Full Adder/1(X)
  AND/1 -> Full Adder/2(Y)
  Full Adder/1(S) -> Sum Out/1
  Y/1 -> AND/2
  X/1 -> AND/1
  Full Adder/2(C) -> C Out/1

== system Multiplier/8-bit_Multiplier/Multiplier/Multiplier Building Block29 ==
  Cin : Inport
  X : Inport  Port=2
  Y : Inport  Port=3
  Sum in : Inport  Port=4
  AND : Logic  IconShape=distinctive  AllPortsSameDT=off  OutDataTypeStr=boolean
  Full Adder : Subsystem
  Sum Out : Outport
  C Out : Outport  Port=2
  wires:
  Cin/1 -> Full Adder/3(Z)
  Sum in/1 -> Full Adder/1(X)
  AND/1 -> Full Adder/2(Y)
  Full Adder/1(S) -> Sum Out/1
  Y/1 -> AND/2
  X/1 -> AND/1
  Full Adder/2(C) -> C Out/1

== system Multiplier/8-bit_Multiplier/Multiplier/Multiplier Building Block3 ==
  Cin : Inport
  X : Inport  Port=2
  Y : Inport  Port=3
  Sum in : Inport  Port=4
  AND : Logic  IconShape=distinctive  AllPortsSameDT=off  OutDataTypeStr=boolean
  Full Adder : Subsystem
  Sum Out : Outport
  C Out : Outport  Port=2
  wires:
  Cin/1 -> Full Adder/3(Z)
  Sum in/1 -> Full Adder/1(X)
  AND/1 -> Full Adder/2(Y)
  Full Adder/1(S) -> Sum Out/1
  Y/1 -> AND/2
  X/1 -> AND/1
  Full Adder/2(C) -> C Out/1

== system Multiplier/8-bit_Multiplier/Multiplier/Multiplier Building Block30 ==
  Cin : Inport
  X : Inport  Port=2
  Y : Inport  Port=3
  Sum in : Inport  Port=4
  AND : Logic  IconShape=distinctive  AllPortsSameDT=off  OutDataTypeStr=boolean
  Full Adder : Subsystem
  Sum Out : Outport
  C Out : Outport  Port=2
  wires:
  Cin/1 -> Full Adder/3(Z)
  Sum in/1 -> Full Adder/1(X)
  AND/1 -> Full Adder/2(Y)
  Full Adder/1(S) -> Sum Out/1
  Y/1 -> AND/2
  X/1 -> AND/1
  Full Adder/2(C) -> C Out/1

== system Multiplier/8-bit_Multiplier/Multiplier/Multiplier Building Block31 ==
  Cin : Inport
  X : Inport  Port=2
  Y : Inport  Port=3
  Sum in : Inport  Port=4
  AND : Logic  IconShape=distinctive  AllPortsSameDT=off  OutDataTypeStr=boolean
  Full Adder : Subsystem
  Sum Out : Outport
  C Out : Outport  Port=2
  wires:
  Cin/1 -> Full Adder/3(Z)
  Sum in/1 -> Full Adder/1(X)
  AND/1 -> Full Adder/2(Y)
  Full Adder/1(S) -> Sum Out/1
  Y/1 -> AND/2
  X/1 -> AND/1
  Full Adder/2(C) -> C Out/1

== system Multiplier/8-bit_Multiplier/Multiplier/Multiplier Building Block32 ==
  Cin : Inport
  X : Inport  Port=2
  Y : Inport  Port=3
  Sum in : Inport  Port=4
  AND : Logic  IconShape=distinctive  AllPortsSameDT=off  OutDataTypeStr=boolean
  Full Adder : Subsystem
  Sum Out : Outport
  C Out : Outport  Port=2
  wires:
  Cin/1 -> Full Adder/3(Z)
  Sum in/1 -> Full Adder/1(X)
  AND/1 -> Full Adder/2(Y)
  Full Adder/1(S) -> Sum Out/1
  Y/1 -> AND/2
  X/1 -> AND/1
  Full Adder/2(C) -> C Out/1

== system Multiplier/8-bit_Multiplier/Multiplier/Multiplier Building Block33 ==
  Cin : Inport
  X : Inport  Port=2
  Y : Inport  Port=3
  Sum in : Inport  Port=4
  AND : Logic  IconShape=distinctive  AllPortsSameDT=off  OutDataTypeStr=boolean
  Full Adder : Subsystem
  Sum Out : Outport
  C Out : Outport  Port=2
  wires:
  Cin/1 -> Full Adder/3(Z)
  Sum in/1 -> Full Adder/1(X)
  AND/1 -> Full Adder/2(Y)
  Full Adder/1(S) -> Sum Out/1
  Y/1 -> AND/2
  X/1 -> AND/1
  Full Adder/2(C) -> C Out/1

== system Multiplier/8-bit_Multiplier/Multiplier/Multiplier Building Block34 ==
  Cin : Inport
  X : Inport  Port=2
  Y : Inport  Port=3
  Sum in : Inport  Port=4
  AND : Logic  IconShape=distinctive  AllPortsSameDT=off  OutDataTypeStr=boolean
  Full Adder : Subsystem
  Sum Out : Outport
  C Out : Outport  Port=2
  wires:
  Cin/1 -> Full Adder/3(Z)
  Sum in/1 -> Full Adder/1(X)
  AND/1 -> Full Adder/2(Y)
  Full Adder/1(S) -> Sum Out/1
  Y/1 -> AND/2
  X/1 -> AND/1
  Full Adder/2(C) -> C Out/1

== system Multiplier/8-bit_Multiplier/Multiplier/Multiplier Building Block35 ==
  Cin : Inport
  X : Inport  Port=2
  Y : Inport  Port=3
  Sum in : Inport  Port=4
  AND : Logic  IconShape=distinctive  AllPortsSameDT=off  OutDataTypeStr=boolean
  Full Adder : Subsystem
  Sum Out : Outport
  C Out : Outport  Port=2
  wires:
  Cin/1 -> Full Adder/3(Z)
  Sum in/1 -> Full Adder/1(X)
  AND/1 -> Full Adder/2(Y)
  Full Adder/1(S) -> Sum Out/1
  Y/1 -> AND/2
  X/1 -> AND/1
  Full Adder/2(C) -> C Out/1

== system Multiplier/8-bit_Multiplier/Multiplier/Multiplier Building Block36 ==
  Cin : Inport
  X : Inport  Port=2
  Y : Inport  Port=3
  Sum in : Inport  Port=4
  AND : Logic  IconShape=distinctive  AllPortsSameDT=off  OutDataTypeStr=boolean
  Full Adder : Subsystem
  Sum Out : Outport
  C Out : Outport  Port=2
  wires:
  Cin/1 -> Full Adder/3(Z)
  Sum in/1 -> Full Adder/1(X)
  AND/1 -> Full Adder/2(Y)
  Full Adder/1(S) -> Sum Out/1
  Y/1 -> AND/2
  X/1 -> AND/1
  Full Adder/2(C) -> C Out/1

== system Multiplier/8-bit_Multiplier/Multiplier/Multiplier Building Block37 ==
  Cin : Inport
  X : Inport  Port=2
  Y : Inport  Port=3
  Sum in : Inport  Port=4
  AND : Logic  IconShape=distinctive  AllPortsSameDT=off  OutDataTypeStr=boolean
  Full Adder : Subsystem
  Sum Out : Outport
  C Out : Outport  Port=2
  wires:
  Cin/1 -> Full Adder/3(Z)
  Sum in/1 -> Full Adder/1(X)
  AND/1 -> Full Adder/2(Y)
  Full Adder/1(S) -> Sum Out/1
  Y/1 -> AND/2
  X/1 -> AND/1
  Full Adder/2(C) -> C Out/1

== system Multiplier/8-bit_Multiplier/Multiplier/Multiplier Building Block38 ==
  Cin : Inport
  X : Inport  Port=2
  Y : Inport  Port=3
  Sum in : Inport  Port=4
  AND : Logic  IconShape=distinctive  AllPortsSameDT=off  OutDataTypeStr=boolean
  Full Adder : Subsystem
  Sum Out : Outport
  C Out : Outport  Port=2
  wires:
  Cin/1 -> Full Adder/3(Z)
  Sum in/1 -> Full Adder/1(X)
  AND/1 -> Full Adder/2(Y)
  Full Adder/1(S) -> Sum Out/1
  Y/1 -> AND/2
  X/1 -> AND/1
  Full Adder/2(C) -> C Out/1

== system Multiplier/8-bit_Multiplier/Multiplier/Multiplier Building Block39 ==
  Cin : Inport
  X : Inport  Port=2
  Y : Inport  Port=3
  Sum in : Inport  Port=4
  AND : Logic  IconShape=distinctive  AllPortsSameDT=off  OutDataTypeStr=boolean
  Full Adder : Subsystem
  Sum Out : Outport
  C Out : Outport  Port=2
  wires:
  Cin/1 -> Full Adder/3(Z)
  Sum in/1 -> Full Adder/1(X)
  AND/1 -> Full Adder/2(Y)
  Full Adder/1(S) -> Sum Out/1
  Y/1 -> AND/2
  X/1 -> AND/1
  Full Adder/2(C) -> C Out/1

== system Multiplier/8-bit_Multiplier/Multiplier/Multiplier Building Block4 ==
  Cin : Inport
  X : Inport  Port=2
  Y : Inport  Port=3
  Sum in : Inport  Port=4
  AND : Logic  IconShape=distinctive  AllPortsSameDT=off  OutDataTypeStr=boolean
  Full Adder : Subsystem
  Sum Out : Outport
  C Out : Outport  Port=2
  wires:
  Cin/1 -> Full Adder/3(Z)
  Sum in/1 -> Full Adder/1(X)
  AND/1 -> Full Adder/2(Y)
  Full Adder/1(S) -> Sum Out/1
  Y/1 -> AND/2
  X/1 -> AND/1
  Full Adder/2(C) -> C Out/1

== system Multiplier/8-bit_Multiplier/Multiplier/Multiplier Building Block40 ==
  Cin : Inport
  X : Inport  Port=2
  Y : Inport  Port=3
  Sum in : Inport  Port=4
  AND : Logic  IconShape=distinctive  AllPortsSameDT=off  OutDataTypeStr=boolean
  Full Adder : Subsystem
  Sum Out : Outport
  C Out : Outport  Port=2
  wires:
  Cin/1 -> Full Adder/3(Z)
  Sum in/1 -> Full Adder/1(X)
  AND/1 -> Full Adder/2(Y)
  Full Adder/1(S) -> Sum Out/1
  Y/1 -> AND/2
  X/1 -> AND/1
  Full Adder/2(C) -> C Out/1

== system Multiplier/8-bit_Multiplier/Multiplier/Multiplier Building Block41 ==
  Cin : Inport
  X : Inport  Port=2
  Y : Inport  Port=3
  Sum in : Inport  Port=4
  AND : Logic  IconShape=distinctive  AllPortsSameDT=off  OutDataTypeStr=boolean
  Full Adder : Subsystem
  Sum Out : Outport
  C Out : Outport  Port=2
  wires:
  Cin/1 -> Full Adder/3(Z)
  Sum in/1 -> Full Adder/1(X)
  AND/1 -> Full Adder/2(Y)
  Full Adder/1(S) -> Sum Out/1
  Y/1 -> AND/2
  X/1 -> AND/1
  Full Adder/2(C) -> C Out/1

== system Multiplier/8-bit_Multiplier/Multiplier/Multiplier Building Block42 ==
  Cin : Inport
  X : Inport  Port=2
  Y : Inport  Port=3
  Sum in : Inport  Port=4
  AND : Logic  IconShape=distinctive  AllPortsSameDT=off  OutDataTypeStr=boolean
  Full Adder : Subsystem
  Sum Out : Outport
  C Out : Outport  Port=2
  wires:
  Cin/1 -> Full Adder/3(Z)
  Sum in/1 -> Full Adder/1(X)
  AND/1 -> Full Adder/2(Y)
  Full Adder/1(S) -> Sum Out/1
  Y/1 -> AND/2
  X/1 -> AND/1
  Full Adder/2(C) -> C Out/1

== system Multiplier/8-bit_Multiplier/Multiplier/Multiplier Building Block43 ==
  Cin : Inport
  X : Inport  Port=2
  Y : Inport  Port=3
  Sum in : Inport  Port=4
  AND : Logic  IconShape=distinctive  AllPortsSameDT=off  OutDataTypeStr=boolean
  Full Adder : Subsystem
  Sum Out : Outport
  C Out : Outport  Port=2
  wires:
  Cin/1 -> Full Adder/3(Z)
  Sum in/1 -> Full Adder/1(X)
  AND/1 -> Full Adder/2(Y)
  Full Adder/1(S) -> Sum Out/1
  Y/1 -> AND/2
  X/1 -> AND/1
  Full Adder/2(C) -> C Out/1

== system Multiplier/8-bit_Multiplier/Multiplier/Multiplier Building Block44 ==
  Cin : Inport
  X : Inport  Port=2
  Y : Inport  Port=3
  Sum in : Inport  Port=4
  AND : Logic  IconShape=distinctive  AllPortsSameDT=off  OutDataTypeStr=boolean
  Full Adder : Subsystem
  Sum Out : Outport
  C Out : Outport  Port=2
  wires:
  Cin/1 -> Full Adder/3(Z)
  Sum in/1 -> Full Adder/1(X)
  AND/1 -> Full Adder/2(Y)
  Full Adder/1(S) -> Sum Out/1
  Y/1 -> AND/2
  X/1 -> AND/1
  Full Adder/2(C) -> C Out/1

== system Multiplier/8-bit_Multiplier/Multiplier/Multiplier Building Block45 ==
  Cin : Inport
  X : Inport  Port=2
  Y : Inport  Port=3
  Sum in : Inport  Port=4
  AND : Logic  IconShape=distinctive  AllPortsSameDT=off  OutDataTypeStr=boolean
  Full Adder : Subsystem
  Sum Out : Outport
  C Out : Outport  Port=2
  wires:
  Cin/1 -> Full Adder/3(Z)
  Sum in/1 -> Full Adder/1(X)
  AND/1 -> Full Adder/2(Y)
  Full Adder/1(S) -> Sum Out/1
  Y/1 -> AND/2
  X/1 -> AND/1
  Full Adder/2(C) -> C Out/1

== system Multiplier/8-bit_Multiplier/Multiplier/Multiplier Building Block46 ==
  Cin : Inport
  X : Inport  Port=2
  Y : Inport  Port=3
  Sum in : Inport  Port=4
  AND : Logic  IconShape=distinctive  AllPortsSameDT=off  OutDataTypeStr=boolean
  Full Adder : Subsystem
  Sum Out : Outport
  C Out : Outport  Port=2
  wires:
  Cin/1 -> Full Adder/3(Z)
  Sum in/1 -> Full Adder/1(X)
  AND/1 -> Full Adder/2(Y)
  Full Adder/1(S) -> Sum Out/1
  Y/1 -> AND/2
  X/1 -> AND/1
  Full Adder/2(C) -> C Out/1

== system Multiplier/8-bit_Multiplier/Multiplier/Multiplier Building Block47 ==
  Cin : Inport
  X : Inport  Port=2
  Y : Inport  Port=3
  Sum in : Inport  Port=4
  AND : Logic  IconShape=distinctive  AllPortsSameDT=off  OutDataTypeStr=boolean
  Full Adder : Subsystem
  Sum Out : Outport
  C Out : Outport  Port=2
  wires:
  Cin/1 -> Full Adder/3(Z)
  Sum in/1 -> Full Adder/1(X)
  AND/1 -> Full Adder/2(Y)
  Full Adder/1(S) -> Sum Out/1
  Y/1 -> AND/2
  X/1 -> AND/1
  Full Adder/2(C) -> C Out/1

== system Multiplier/8-bit_Multiplier/Multiplier/Multiplier Building Block48 ==
  Cin : Inport
  X : Inport  Port=2
  Y : Inport  Port=3
  Sum in : Inport  Port=4
  AND : Logic  IconShape=distinctive  AllPortsSameDT=off  OutDataTypeStr=boolean
  Full Adder : Subsystem
  Sum Out : Outport
  C Out : Outport  Port=2
  wires:
  Cin/1 -> Full Adder/3(Z)
  Sum in/1 -> Full Adder/1(X)
  AND/1 -> Full Adder/2(Y)
  Full Adder/1(S) -> Sum Out/1
  Y/1 -> AND/2
  X/1 -> AND/1
  Full Adder/2(C) -> C Out/1

== system Multiplier/8-bit_Multiplier/Multiplier/Multiplier Building Block49 ==
  Cin : Inport
  X : Inport  Port=2
  Y : Inport  Port=3
  Sum in : Inport  Port=4
  AND : Logic  IconShape=distinctive  AllPortsSameDT=off  OutDataTypeStr=boolean
  Full Adder : Subsystem
  Sum Out : Outport
  C Out : Outport  Port=2
  wires:
  Cin/1 -> Full Adder/3(Z)
  Sum in/1 -> Full Adder/1(X)
  AND/1 -> Full Adder/2(Y)
  Full Adder/1(S) -> Sum Out/1
  Y/1 -> AND/2
  X/1 -> AND/1
  Full Adder/2(C) -> C Out/1

== system Multiplier/8-bit_Multiplier/Multiplier/Multiplier Building Block5 ==
  Cin : Inport
  X : Inport  Port=2
  Y : Inport  Port=3
  Sum in : Inport  Port=4
  AND : Logic  IconShape=distinctive  AllPortsSameDT=off  OutDataTypeStr=boolean
  Full Adder : Subsystem
  Sum Out : Outport
  C Out : Outport  Port=2
  wires:
  Cin/1 -> Full Adder/3(Z)
  Sum in/1 -> Full Adder/1(X)
  AND/1 -> Full Adder/2(Y)
  Full Adder/1(S) -> Sum Out/1
  Y/1 -> AND/2
  X/1 -> AND/1
  Full Adder/2(C) -> C Out/1

== system Multiplier/8-bit_Multiplier/Multiplier/Multiplier Building Block50 ==
  Cin : Inport
  X : Inport  Port=2
  Y : Inport  Port=3
  Sum in : Inport  Port=4
  AND : Logic  IconShape=distinctive  AllPortsSameDT=off  OutDataTypeStr=boolean
  Full Adder : Subsystem
  Sum Out : Outport
  C Out : Outport  Port=2
  wires:
  Cin/1 -> Full Adder/3(Z)
  Sum in/1 -> Full Adder/1(X)
  AND/1 -> Full Adder/2(Y)
  Full Adder/1(S) -> Sum Out/1
  Y/1 -> AND/2
  X/1 -> AND/1
  Full Adder/2(C) -> C Out/1

== system Multiplier/8-bit_Multiplier/Multiplier/Multiplier Building Block51 ==
  Cin : Inport
  X : Inport  Port=2
  Y : Inport  Port=3
  Sum in : Inport  Port=4
  AND : Logic  IconShape=distinctive  AllPortsSameDT=off  OutDataTypeStr=boolean
  Full Adder : Subsystem
  Sum Out : Outport
  C Out : Outport  Port=2
  wires:
  Cin/1 -> Full Adder/3(Z)
  Sum in/1 -> Full Adder/1(X)
  AND/1 -> Full Adder/2(Y)
  Full Adder/1(S) -> Sum Out/1
  Y/1 -> AND/2
  X/1 -> AND/1
  Full Adder/2(C) -> C Out/1

== system Multiplier/8-bit_Multiplier/Multiplier/Multiplier Building Block52 ==
  Cin : Inport
  X : Inport  Port=2
  Y : Inport  Port=3
  Sum in : Inport  Port=4
  AND : Logic  IconShape=distinctive  AllPortsSameDT=off  OutDataTypeStr=boolean
  Full Adder : Subsystem
  Sum Out : Outport
  C Out : Outport  Port=2
  wires:
  Cin/1 -> Full Adder/3(Z)
  Sum in/1 -> Full Adder/1(X)
  AND/1 -> Full Adder/2(Y)
  Full Adder/1(S) -> Sum Out/1
  Y/1 -> AND/2
  X/1 -> AND/1
  Full Adder/2(C) -> C Out/1

== system Multiplier/8-bit_Multiplier/Multiplier/Multiplier Building Block53 ==
  Cin : Inport
  X : Inport  Port=2
  Y : Inport  Port=3
  Sum in : Inport  Port=4
  AND : Logic  IconShape=distinctive  AllPortsSameDT=off  OutDataTypeStr=boolean
  Full Adder : Subsystem
  Sum Out : Outport
  C Out : Outport  Port=2
  wires:
  Cin/1 -> Full Adder/3(Z)
  Sum in/1 -> Full Adder/1(X)
  AND/1 -> Full Adder/2(Y)
  Full Adder/1(S) -> Sum Out/1
  Y/1 -> AND/2
  X/1 -> AND/1
  Full Adder/2(C) -> C Out/1
